simulink model "Final_Project_v3b"  (R2013a)
settings: Solver=ode45  StartTime=0.0  StopTime=inf  RelTol=1e-3
InitFcn:
  | start_EEVSCube2
  | 
  | %links masses
  | 
  | m=20;%Kg
  | 
  | l=1;%meter
  | 
  | %controls
  | 
  | a=0.3; %singularity positive gain
  | 
  | %Chaser
  | 
  | lb=1;%meter distance 1joint to CM
  | 
  | %Target
  | 
  | mt=5;%kg target mass
  | lt=1;%meter  side lenght
  | It=(1/6)*(lt^2);
  | 
  | %Target Initial Conitions
  | 
  | x_t=2;
  | y_t=3;
  | theta_t=0.7853;
  | 
  | Init_t=[x_t;y_t;theta_t];
undefined symbols (not defined in the file or in its folder): mesh_A, mesh_B
libraries: vrlib x2, dspinverses x1, aerolibanimutils x1
(part 1 of 2)
settings Model: Creator=Grompone  LastModifiedBy=Grompone

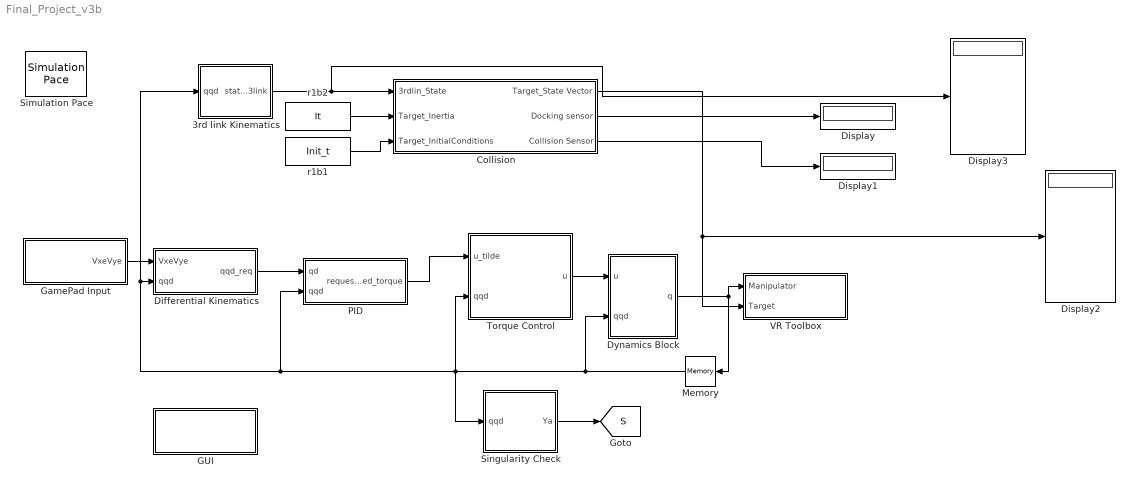
== system Final_Project_v3b ==
  3rd link Kinematics : MATLAB Function  TreatAsAtomicUnit=on
  Collision : Subsystem
  Differential Kinematics : Subsystem
  Display{,1..3} (4 alike) : Display
  Dynamics Block : Subsystem
  GUI : Subsystem
  GamePad Input : Subsystem
  Memory : Memory  X0=[0 0 0 0 0 0 0 0 0]'
  PID : Subsystem
  Simulation Pace : aerolibanimutils/Simulation Pace  SimulationPace=1  SleepMode=MATLAB Thread  OutputPaceError=off  SampleTime=1/30
      settings: AttributesFormatString=%<SimulationPace> sec/sec
  Singularity Check : MATLAB Function  TreatAsAtomicUnit=on
  Torque Control : Subsystem
  VR Toolbox : Subsystem
  r1b1 : Constant  Value=Init_t
  r1b2 : Constant  Value=It
  tag scope: S=global
  wires:
  Torque Control/1(u) -> Dynamics Block/1(u)
  PID/1(requested_torque) -> Torque Control/1(u_tilde)
  Dynamics Block/1(q) -> VR Toolbox/1(Manipulator), Memory/1
  Differential Kinematics/1(qqd_req) -> PID/1(qd)
  GamePad Input/1(VxeVye) -> Differential Kinematics/1(VxeVye)
  Memory/1 -> Dynamics Block/2(qqd), Torque Control/2(qqd), Singularity Check/1(qqd), PID/2(qqd), 3rd link Kinematics/1(qqd), Differential Kinematics/2(qqd)
  Singularity Check/1(Ya) -> [S]
  r1b2/1 -> Collision/2(Target_Inertia)
  r1b1/1 -> Collision/3(Target_InitialConditions)
  Collision/1(Target_State Vector) -> Display2/1, VR Toolbox/2(Target)
  3rd link Kinematics/1(state_3link) -> Display3/1, Collision/1(3rdlin_State)
  Collision/2(Docking sensor) -> Display/1
  Collision/3(Collision Sensor) -> Display1/1

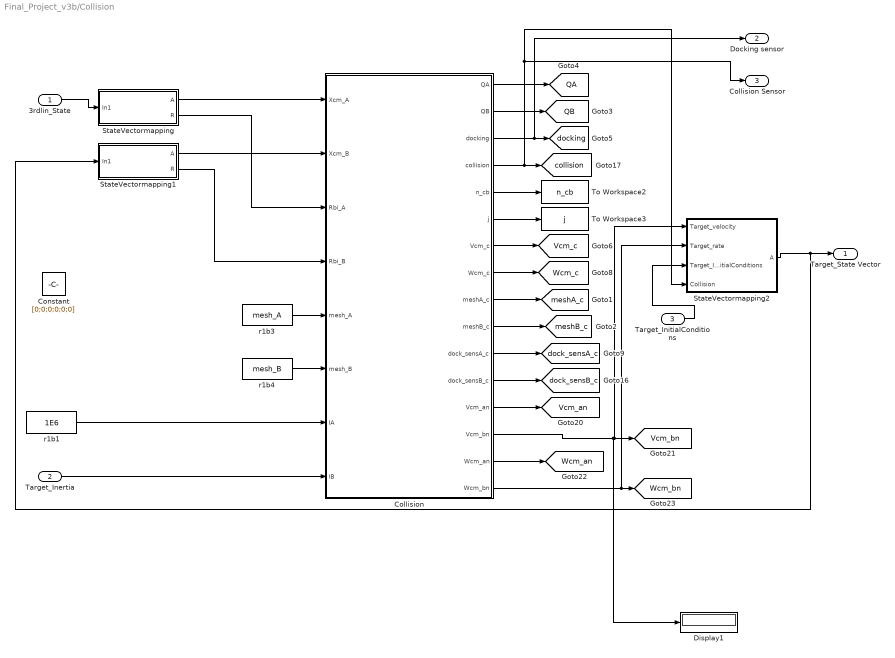
== system Final_Project_v3b/Collision ==
  3rdlin_State : Inport
  Target_Inertia : Inport  Port=2
  Target_InitialConditions : Inport  Port=3
  Collision : Subsystem  mask{mA=1e6, mB=mt, sigma=0.01, sigma_dock=0.1, dotsigma_dock=1, dock_sensA=[0.5 0 0]', dock_sensB=[-0.5 0 0]', epsilon=1}
      mask prompts: mA "Mass of body A [Kg]"; mB "Mass of body B [Kg]"; sigma "Minimum distance for contact [m]"; sigma_dock "Minimum distance for docking (must be greater than contact distance) [m]"; dotsigma_dock "Maximum relative velocity for docking [m/s]"; dock_sensA "Docking sensor position (Body RF) on body A (as [x y z]') [m]"; dock_sensB "Docking sensor position (Body RF) on body B (as [x y z]') [m]"; epsilon "Coefficent of restitution"
      mask help: This block implements collision detection and responce for two rigid bodies of general shapes.
      mask init:
      | ma_mb = [mA; 
      |          mB];
      mask Display:
      | image(imread('collision.jpeg'))
      | color('red');
      | disp('Collision \n Detection and Responce \n v.1.0.9')
      | port_label('input',1,'Xcm_A')
      | port_label('input',2,'Xcm_B')
      | port_label('input',3,'Rbi_A')
      | port_label('input',4,'Rbi_B')
      | port_label('input',5,'mesh_A')
      | port_label('input',6,'mesh_B')
      | port_label('input',7,'IA')
      | port_label('input',8,'IB')
      | 
      | port_label('output',1,'QA')
      | port_label('output',2,'QB')
      | port_label('output',3,'docking')
      | port_label('output',4,'collision')
      | port_label('output',5,'n_cb')
      | port_label('output',6,'j')
      | port_label('output',7,'Vcm_c')
      | port_label('output',8,'Wcm_c')
      | port_label('output',9,'meshA_c')
      | port_label('output',10,'meshB_c')
      | port_label('output',11,'dock_sensA_c')
      | port_label('output',12,'dock_sensB_c')
      | port_label('output',13,'Vcm_an')
      | port_label('output',14,'Vcm_bn')
      | port_label('output',15,'Wcm_an')
      | port_label('output',16,'Wcm_bn')
  Constant : Constant  Value=[0;0;0;0;0;0]
  Display1 : Display
  StateVectormapping : Subsystem
  StateVectormapping1 : Subsystem
  StateVectormapping2 : Subsystem
  To Workspace2 : ToWorkspace  VariableName=n_cb  SampleTime=-1
  To Workspace3 : ToWorkspace  VariableName=j  SampleTime=-1
  r1b1 : Constant  Value=1E6
  r1b3 : Constant  Value=mesh_A
  r1b4 : Constant  Value=mesh_B
  Target_State Vector : Outport
  Docking sensor : Outport  Port=2
  Collision Sensor : Outport  Port=3
  tag scope: QA=global, QB=global, Vcm_an=global, Vcm_bn=global, Vcm_c=global, Wcm_an=global, Wcm_bn=global, Wcm_c=global, collision=global, dock_sensA_c=global, dock_sensB_c=global, docking=global, meshA_c=global, meshB_c=global
  wires:
  Collision/1(QA) -> [QA]
  Collision/2(QB) -> [QB]
  Collision/3(docking) -> Docking sensor/1, [docking]
  Collision/6(j) -> To Workspace3/1
  Collision/4(collision) -> StateVectormapping2/4(Collision), Collision Sensor/1, [collision]
  StateVectormapping/2(R) -> Collision/3(Rbi_A)
  StateVectormapping1/2(R) -> Collision/4(Rbi_B)
  r1b3/1 -> Collision/5(mesh_A)
  r1b4/1 -> Collision/6(mesh_B)
  Collision/5(n_cb) -> To Workspace2/1
  Collision/7(Vcm_c) -> [Vcm_c]
  Collision/8(Wcm_c) -> [Wcm_c]
  Collision/9(meshA_c) -> [meshA_c]
  Collision/10(meshB_c) -> [meshB_c]
  Collision/11(dock_sensA_c) -> [dock_sensA_c]
  Collision/12(dock_sensB_c) -> [dock_sensB_c]
  r1b1/1 -> Collision/7(IA)
  Collision/13(Vcm_an) -> [Vcm_an]
  Collision/15(Wcm_an) -> [Wcm_an]
  Collision/16(Wcm_bn) -> StateVectormapping2/2(Target_rate), [Wcm_bn]
  3rdlin_State/1 -> StateVectormapping/1(In1)
  StateVectormapping1/1(A) -> Collision/2(Xcm_B)
  Collision/14(Vcm_bn) -> Display1/1, StateVectormapping2/1(Target_velocity), [Vcm_bn]
  Target_InitialConditions/1 -> StateVectormapping2/3(Target_InitialConditions)
  Target_Inertia/1 -> Collision/8(IB)
  StateVectormapping/1(A) -> Collision/1(Xcm_A)
  StateVectormapping2/1(A) -> StateVectormapping1/1(In1), Target_State Vector/1

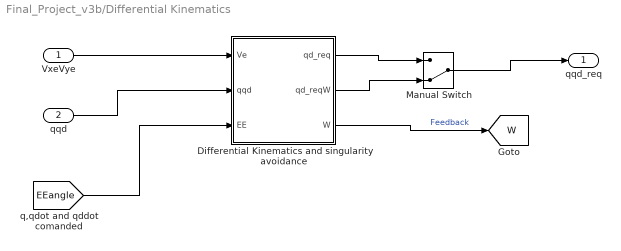
== system Final_Project_v3b/Differential Kinematics ==
  VxeVye : Inport
  qqd : Inport  Port=2
  Differential Kinematics and singularity avoidance : MATLAB Function  TreatAsAtomicUnit=on
  Manual Switch : ManualSwitch  CurrentSetting=0
  qqd_req : Outport
  tag scope: W=global
  wires:
  VxeVye/1 -> Differential Kinematics and singularity avoidance/1(Ve)
  qqd/1 -> Differential Kinematics and singularity avoidance/2(qqd)
  Differential Kinematics and singularity avoidance/3(W) -> [W]  "Feedback"
  Differential Kinematics and singularity avoidance/1(qd_req) -> Manual Switch/1
  Differential Kinematics and singularity avoidance/2(qd_reqW) -> Manual Switch/2
  Manual Switch/1 -> qqd_req/1
  [EEangle] -> Differential Kinematics and singularity avoidance/3(EE)

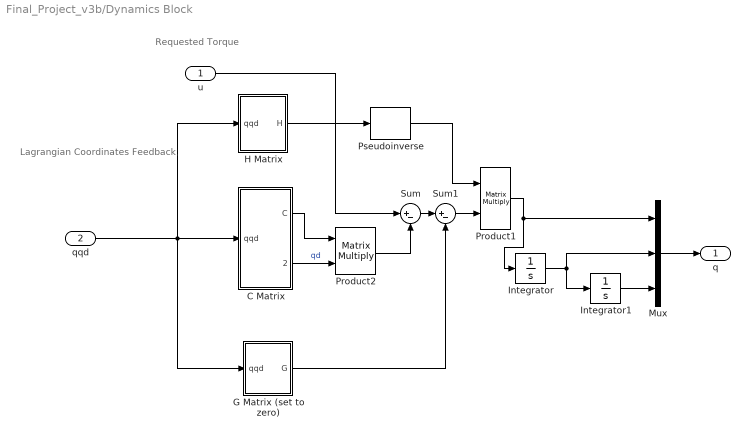
== system Final_Project_v3b/Dynamics Block ==
  note: Requested Torque
  note: Lagrangian Coordinates Feedback
  u : Inport
  qqd : Inport  Port=2
  C Matrix : MATLAB Function  TreatAsAtomicUnit=on
  G Matrix (set to zero) : MATLAB Function  TreatAsAtomicUnit=on
  H Matrix : MATLAB Function  TreatAsAtomicUnit=on
  Integrator : Integrator  InitialCondition=[0;0;0]
  Integrator1 : Integrator  InitialCondition=[0;0;0]
  Mux : Mux  Inputs=3
  Product1 : Product  Multiplication=Matrix(*)
  Product2 : Product  Multiplication=Matrix(*)  OutDataTypeStr=int8  LockScale=on
  Pseudoinverse : dspinverses/Pseudoinverse  wanterr=off
  Sum : Sum  Inputs=|+-
  Sum1 : Sum  Inputs=|+-
  q : Outport
  wires:
  Integrator/1 -> Mux/2, Integrator1/1
  Integrator1/1 -> Mux/3
  Mux/1 -> q/1
  C Matrix/1(C) -> Product2/1
  H Matrix/1(H) -> Pseudoinverse/1
  Pseudoinverse/1 -> Product1/1
  Product1/1 -> Mux/1, Integrator/1
  Sum/1 -> Sum1/1
  Sum1/1 -> Product1/2
  G Matrix (set to zero)/1(G) -> Sum1/2
  Product2/1 -> Sum/2
  u/1 -> Sum/1
  C Matrix/2(q_dot) -> Product2/2  "qd"
  qqd/1 -> G Matrix (set to zero)/1(qqd), H Matrix/1(qqd), C Matrix/1(qqd)

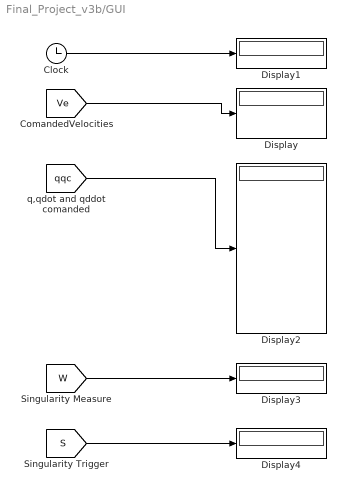
== system Final_Project_v3b/GUI ==
  Clock : Clock
  Display{,1..4} (5 alike) : Display
  wires:
  [Ve] -> Display/1
  Clock/1 -> Display1/1
  [qqc] -> Display2/1
  [W] -> Display3/1
  [S] -> Display4/1

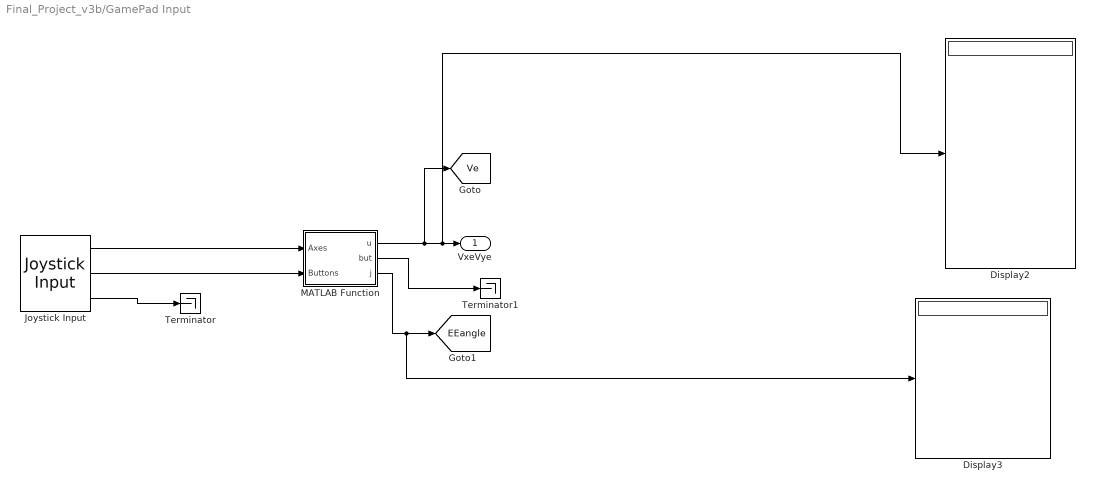
== system Final_Project_v3b/GamePad Input ==
  Display2 : Display
  Display3 : Display
  Joystick Input : vrlib/Joystick Input  joyid=1  adjustports=on  forcefeed=off
  MATLAB Function : MATLAB Function  TreatAsAtomicUnit=on
  Terminator : Terminator
  Terminator1 : Terminator
  VxeVye : Outport
  tag scope: EEangle=global, Ve=global
  wires:
  Joystick Input/1 -> MATLAB Function/1(Axes)
  Joystick Input/2 -> MATLAB Function/2(Buttons)
  MATLAB Function/1(u) -> [Ve], Display2/1, VxeVye/1
  Joystick Input/3 -> Terminator/1
  MATLAB Function/2(but) -> Terminator1/1
  MATLAB Function/3(j) -> Display3/1, [EEangle]

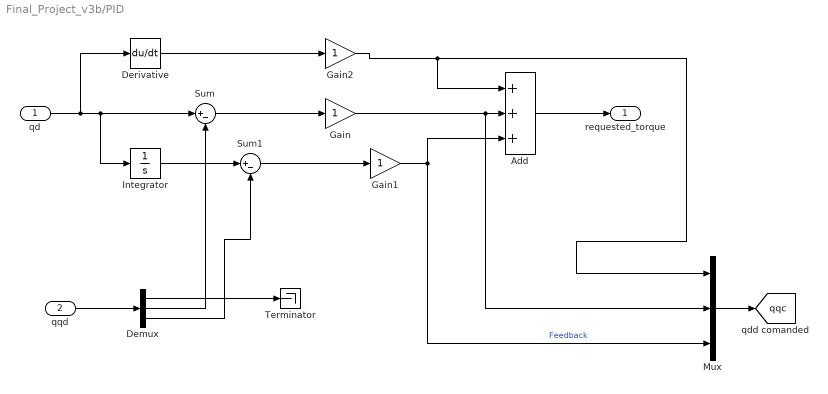
== system Final_Project_v3b/PID ==
  qd : Inport
  qqd : Inport  Port=2
  Add : Sum  Inputs=+++
  Demux : Demux  Outputs=3
  Derivative : Derivative
  Gain : Gain
  Gain1 : Gain
  Gain2 : Gain
  Integrator : Integrator  InitialCondition=[0; 0; 0]
  Mux : Mux  Inputs=3
  Sum : Sum  Inputs=|+-
  Sum1 : Sum  Inputs=|+-
  Terminator : Terminator
  requested_torque : Outport
  tag scope: qqc=global
  wires:
  qqd/1 -> Demux/1
  Demux/2 -> Sum/2
  Demux/1 -> Terminator/1
  Sum/1 -> Gain/1
  qd/1 -> Derivative/1, Integrator/1, Sum/1
  Gain/1 -> Mux/2, Add/2
  Sum1/1 -> Gain1/1
  Demux/3 -> Sum1/2
  Add/1 -> requested_torque/1
  Mux/1 -> [qqc]
  Gain1/1 -> Mux/3, Add/3  "Feedback"
  Integrator/1 -> Sum1/1
  Gain2/1 -> Add/1, Mux/1
  Derivative/1 -> Gain2/1

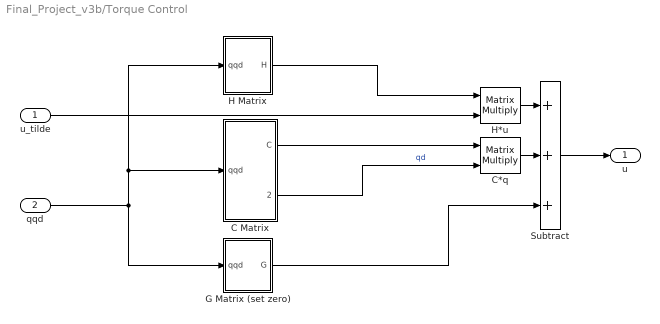
== system Final_Project_v3b/Torque Control ==
  u_tilde : Inport
  qqd : Inport  Port=2
  C Matrix : MATLAB Function  TreatAsAtomicUnit=on
  C*q : Product  Multiplication=Matrix(*)
  G Matrix (set zero) : MATLAB Function  TreatAsAtomicUnit=on
  H Matrix : MATLAB Function  TreatAsAtomicUnit=on
  H*u : Product  Multiplication=Matrix(*)
  Subtract : Sum  Inputs=+++
  u : Outport
  wires:
  H*u/1 -> Subtract/1
  Subtract/1 -> u/1
  C*q/1 -> Subtract/2
  C Matrix/1(C) -> C*q/1
  G Matrix (set zero)/1(G) -> Subtract/3
  C Matrix/2(q_dot) -> C*q/2  "qd"
  u_tilde/1 -> H*u/2
  H Matrix/1(H) -> H*u/1
  qqd/1 -> H Matrix/1(qqd), C Matrix/1(qqd), G Matrix (set zero)/1(qqd)

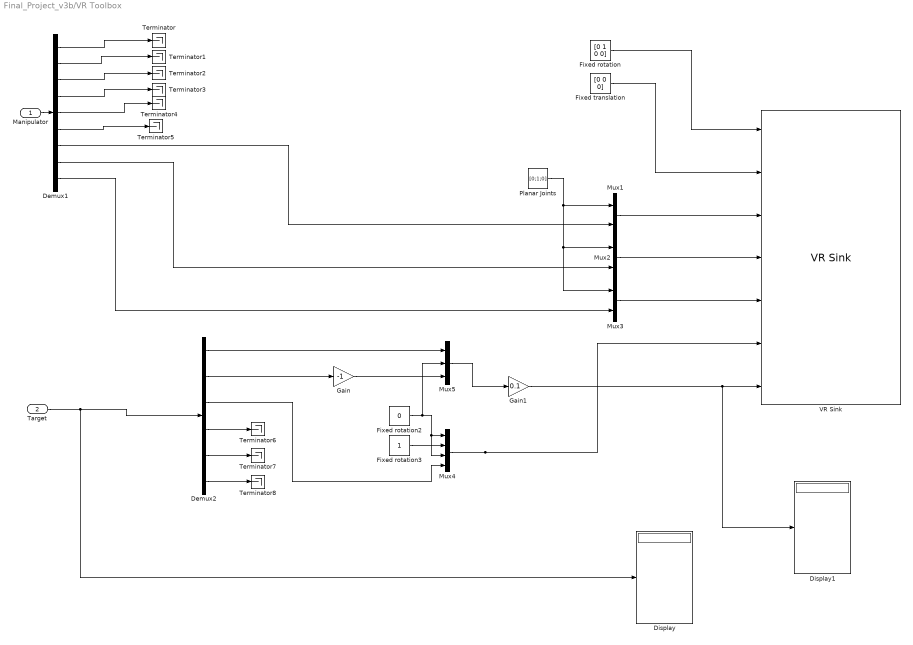
== system Final_Project_v3b/VR Toolbox ==
  Manipulator : Inport
  Target : Inport  Port=2
  Demux1 : Demux  Outputs=9
  Demux2 : Demux  Outputs=6
  Display : Display
  Display1 : Display
  Fixed rotation : Constant  Value=[0 1 0 0]
  Fixed rotation2 : Constant  Value=0
  Fixed rotation3 : Constant
  Fixed translation : Constant  Value=[0 0 0]
  Gain : Gain  Gain=-1
  Gain1 : Gain  Gain=0.1
  Mux1 : Mux  Inputs=2
  Mux2 : Mux  Inputs=2
  Mux3 : Mux  Inputs=2
  Mux4 : Mux
  Mux5 : Mux  Inputs=3
  Planar Joints : Constant  Value=[0;1;0]
  Terminator{,1..8} (9 alike) : Terminator
  VR Sink : vrlib/VR Sink  InstantiateOnLoad=on  SampleTime=0.1  ViewEnable=on  RemoteChange=off  RemoteView=off  FieldsWritten=CHASER.rotation.4.1.1.double#CHASER.translation.3.1.1.double#Joint1.rotation.4.1.1.double#Joint2.rotation.4.1.1.double#Joint3.rotation.4.1.1.double#TARGET.rotation.4.1.1.double#TARGET.translation.3.1.1.double  WorldFileName=final1.wrl  AutoView=off  VideoDimensions=[]  AllowVariableSize=off  FigureProperties="{'Position', 'Name', 'Viewpoint', 'CameraBound', 'CameraDirection', 'CameraPosition', 'CameraUpVector', 'ZoomFactor', 'Antialiasing', 'Headlight', 'Lighting', 'NavPanel', 'StatusBar', 'ToolBar', 'Textures', 'Transparency', 'Triad', 'Wireframe', 'NavZones', 'NavMode', 'NavSpeed', 'CaptureFileFormat', 'CaptureFileName', 'Record2DCompressMethod', 'Record2DCompressQuality', 'Record2D', 'Record2DFileName', 'Record2DFPS'; [5.0000000000000000e+00   9.2000000000000000e+01   5.7600000000000000e+02   3.8000000000000000e+02], '', '_untitled_1', 'on', [0.0000000000000000e+00   0.0000000000000000e+00  -1.0000000000000000e+00], [0.0000000000000000e+00   0.0000000000000000e+00   0.0000000000000000e+00], [0.0000000000000000e+00   1.0000000000000000e+00   0.0000000000000000e+00], [1.0000000000000000e+00], 'on', 'on', 'on', 'halfbar', 'on', 'on', 'on', 'on', 'none', 'off', 'off', 'fly', 'normal', 'tif', '%f_anim_%n.tif', 'auto', [7.5000000000000000e+01], 'off', '%f_anim_%n.avi', [1.5000000000000000e+01]}"
  wires:
  Planar Joints/1 -> Mux3/1, Mux2/1, Mux1/1
  Manipulator/1 -> Demux1/1
  Demux1/8 -> Mux2/2
  Demux1/9 -> Mux3/2
  Demux1/7 -> Mux1/2
  Demux1/1 -> Terminator/1
  Demux1/2 -> Terminator1/1
  Demux1/3 -> Terminator2/1
  Demux1/4 -> Terminator3/1
  Demux1/5 -> Terminator4/1
  Demux1/6 -> Terminator5/1
  Fixed rotation/1 -> VR Sink/1
  Fixed translation/1 -> VR Sink/2
  Mux1/1 -> VR Sink/3
  Mux2/1 -> VR Sink/4
  Mux3/1 -> VR Sink/5
  Target/1 -> Display/1, Demux2/1
  Fixed rotation3/1 -> Mux4/2
  Fixed rotation2/1 -> Mux5/2, Mux4/3, Mux4/1
  Demux2/1 -> Mux5/1
  Demux2/2 -> Gain/1
  Demux2/3 -> Mux4/4
  Demux2/4 -> Terminator6/1
  Demux2/5 -> Terminator7/1
  Demux2/6 -> Terminator8/1
  Gain/1 -> Mux5/3
  Mux4/1 -> VR Sink/6
  Mux5/1 -> Gain1/1
  Gain1/1 -> Display1/1, VR Sink/7

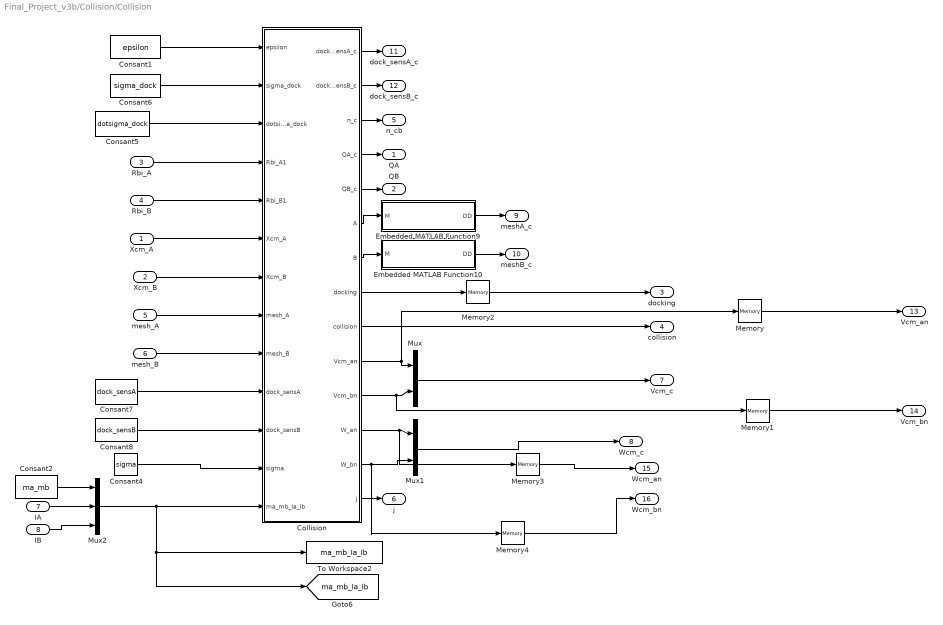
== system Final_Project_v3b/Collision/Collision ==
  Xcm_A : Inport
  Xcm_B : Inport  Port=2
  Rbi_A : Inport  Port=3
  Rbi_B : Inport  Port=4
  mesh_A : Inport  Port=5
  mesh_B : Inport  Port=6
  IA : Inport  Port=7
  IB : Inport  Port=8
  Collision : MATLAB Function  TreatAsAtomicUnit=on
  Consant1 : Constant  Value=epsilon
  Consant2 : Constant  Value=ma_mb
  Consant4 : Constant  Value=sigma
  Consant5 : Constant  Value=dotsigma_dock
  Consant6 : Constant  Value=sigma_dock
  Consant7 : Constant  Value=dock_sensA
  Consant8 : Constant  Value=dock_sensB
  Embedded MATLAB Function10 : MATLAB Function  TreatAsAtomicUnit=on
  Embedded MATLAB Function9 : MATLAB Function  TreatAsAtomicUnit=on
  Memory{,1,3..4} (4 alike) : Memory  X0=zeros(3,1)
  Memory2 : Memory
  Mux : Mux  Inputs=2
  Mux1 : Mux  Inputs=2
  Mux2 : Mux  Inputs=3
  To Workspace2 : ToWorkspace  VariableName=ma_mb_Ia_Ib  SampleTime=-1
  QA : Outport
  QB : Outport  Port=2
  docking : Outport  Port=3
  collision : Outport  Port=4
  n_cb : Outport  Port=5
  j : Outport  Port=6
  Vcm_c : Outport  Port=7
  Wcm_c : Outport  Port=8
  meshA_c : Outport  Port=9
  meshB_c : Outport  Port=10
  dock_sensA_c : Outport  Port=11
  dock_sensB_c : Outport  Port=12
  Vcm_an : Outport  Port=13
  Vcm_bn : Outport  Port=14
  Wcm_an : Outport  Port=15
  Wcm_bn : Outport  Port=16
  tag scope: ma_mb_Ia_Ib=global
  wires:
  Embedded MATLAB Function9/1(DD) -> meshA_c/1
  Embedded MATLAB Function10/1(DD) -> meshB_c/1
  Collision/6(A) -> Embedded MATLAB Function9/1(M)
  Collision/7(B) -> Embedded MATLAB Function10/1(M)
  Rbi_B/1 -> Collision/5(Rbi_B1)
  Xcm_A/1 -> Collision/6(Xcm_A)
  mesh_A/1 -> Collision/8(mesh_A)
  mesh_B/1 -> Collision/9(mesh_B)
  Collision/3(n_c) -> n_cb/1
  Collision/8(docking) -> Memory2/1
  Collision/10(Vcm_an) -> Mux/1, Memory/1
  Collision/13(W_bn) -> Mux1/2, Memory4/1
  Collision/14(j) -> j/1
  Collision/9(collision) -> collision/1
  Mux/1 -> Vcm_c/1
  Mux1/1 -> Wcm_c/1
  Collision/4(QA_c) -> QA/1
  Collision/5(QB_c) -> QB/1
  Collision/11(Vcm_bn) -> Memory1/1, Mux/2
  Collision/12(W_an) -> Memory3/1, Mux1/1
  Xcm_B/1 -> Collision/7(Xcm_B)
  Collision/2(dock_sensB_c) -> dock_sensB_c/1
  Collision/1(dock_sensA_c) -> dock_sensA_c/1
  Consant4/1 -> Collision/12(sigma)
  Consant5/1 -> Collision/3(dotsigma_dock)
  Rbi_A/1 -> Collision/4(Rbi_A1)
  Consant6/1 -> Collision/2(sigma_dock)
  Consant7/1 -> Collision/10(dock_sensA)
  Consant8/1 -> Collision/11(dock_sensB)
  Consant1/1 -> Collision/1(epsilon)
  Mux2/1 -> Collision/13(ma_mb_Ia_Ib), To Workspace2/1, [ma_mb_Ia_Ib]
  Consant2/1 -> Mux2/1
  IA/1 -> Mux2/2
  IB/1 -> Mux2/3
  Memory/1 -> Vcm_an/1
  Memory1/1 -> Vcm_bn/1
  Memory3/1 -> Wcm_an/1
  Memory4/1 -> Wcm_bn/1
  Memory2/1 -> docking/1

== system Final_Project_v3b/Collision/StateVectormapping ==
  In1 : Inport
  Rotation MAtrix1 : MATLAB Function  TreatAsAtomicUnit=on
  A : Outport
  R : Outport  Port=2
  wires:
  Rotation MAtrix1/2(R) -> R/1
  In1/1 -> Rotation MAtrix1/1(u)
  Rotation MAtrix1/1(y) -> A/1

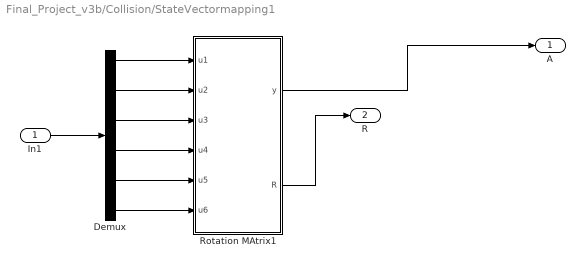
== system Final_Project_v3b/Collision/StateVectormapping1 ==
  In1 : Inport
  Demux : Demux  Outputs=6
  Rotation MAtrix1 : MATLAB Function  TreatAsAtomicUnit=on
  A : Outport  PortDimensions=[9,1]
  R : Outport  Port=2
  wires:
  Demux/1 -> Rotation MAtrix1/1(u1)
  Demux/2 -> Rotation MAtrix1/2(u2)
  Demux/3 -> Rotation MAtrix1/3(u3)
  Demux/6 -> Rotation MAtrix1/6(u6)
  Demux/4 -> Rotation MAtrix1/4(u4)
  Demux/5 -> Rotation MAtrix1/5(u5)
  In1/1 -> Demux/1
  Rotation MAtrix1/2(R) -> R/1
  Rotation MAtrix1/1(y) -> A/1

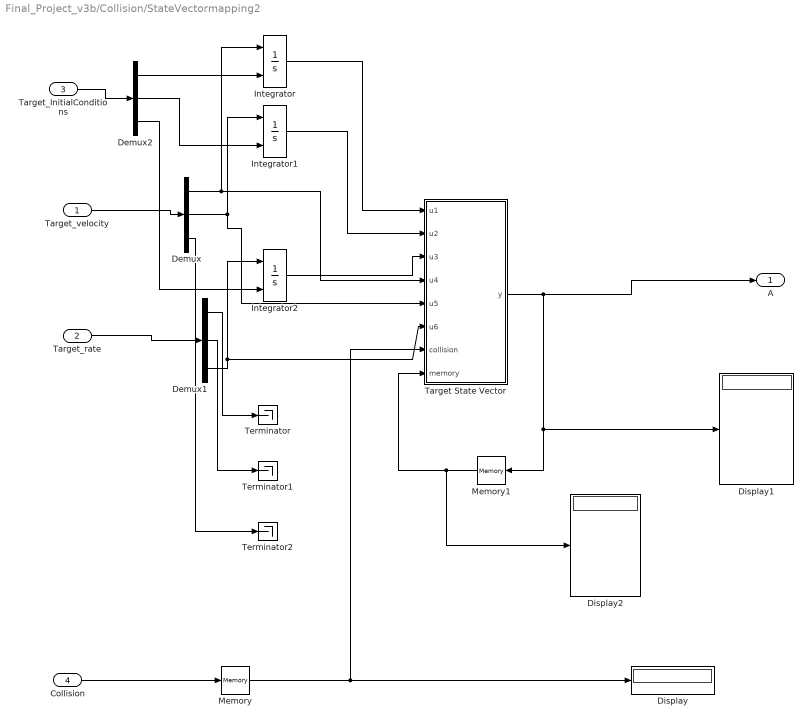
== system Final_Project_v3b/Collision/StateVectormapping2 ==
  Target_velocity : Inport
  Target_rate : Inport  Port=2
  Target_InitialConditions : Inport  Port=3
  Collision : Inport  Port=4
  Demux : Demux  Outputs=3
  Demux1 : Demux  Outputs=3
  Demux2 : Demux  Outputs=3
  Display : Display
  Display1 : Display
  Display2 : Display
  Integrator : Integrator  InitialConditionSource=external
  Integrator1 : Integrator  InitialConditionSource=external
  Integrator2 : Integrator  InitialConditionSource=external
  Memory : Memory  X0=1
  Memory1 : Memory  X0=[0 0 0 0 0 0]'
  Target State Vector : MATLAB Function  TreatAsAtomicUnit=on
  Terminator : Terminator
  Terminator1 : Terminator
  Terminator2 : Terminator
  A : Outport
  wires:
  Target_velocity/1 -> Demux/1
  Target_rate/1 -> Demux1/1
  Demux1/3 -> Integrator2/1, Target State Vector/6(u6)
  Demux/2 -> Target State Vector/5(u5), Integrator1/1
  Demux/1 -> Target State Vector/4(u4), Integrator/1
  Integrator/1 -> Target State Vector/1(u1)
  Integrator1/1 -> Target State Vector/2(u2)
  Integrator2/1 -> Target State Vector/3(u3)
  Demux1/2 -> Terminator1/1
  Demux1/1 -> Terminator/1
  Target_InitialConditions/1 -> Demux2/1
  Demux2/1 -> Integrator/2
  Demux2/2 -> Integrator1/2
  Demux2/3 -> Integrator2/2
  Demux/3 -> Terminator2/1
  Target State Vector/1(y) -> Display1/1, Memory1/1, A/1
  Collision/1 -> Memory/1
  Memory1/1 -> Display2/1, Target State Vector/8(memory)
  Memory/1 -> Target State Vector/7(collision), Display/1

== matlab function Final_Project_v3b/Dynamics Block/C Matrix ==
  data: qqd input; C output; m parameter; l parameter; q_dot output
function [C,q_dot] = fcn(qqd,m,l)
q=[qqd(7); qqd(8); qqd(9)];
q_dot=[qqd(4); qqd(5); qqd(6)];
C=[                                                                                                                                                                                                                                                                                                                                                                                                                                                                                                                                                  (m*abs(l)^2*(2*sin(conj(q(1))) + sin(conj(q(1)) + conj(q(2)) + conj(q(3))) + 2*sin(conj(q(1)) + conj(q(2))))*(cos(q(1) + q(2) + q(3))*(q_dot(1) + q_dot(2) + q_dot(3)) + 2*cos(q(1) + q(2))*(q_dot(1) + q_dot(2)) + 2*q_dot(1)*cos(q(1))))/8 - (m*abs(l)^2*(2*cos(conj(q(1))) + cos(conj(q(1)) + conj(q(2)) + conj(q(3))) + 2*cos(conj(q(1)) + conj(q(2))))*(sin(q(1) + q(2) + q(3))*(q_dot(1) + q_dot(2) + q_dot(3)) + 2*sin(q(1) + q(2))*(q_dot(1) + q_dot(2)) + 2*q_dot(1)*sin(q(1))))/8 + (m*abs(l)^2*(cos(q(1) + q(2))*(q_dot(1) + q_dot(2)) + 2*q_dot(1)*cos(q(1)))*(2*sin(conj(q(1))) + sin(conj(q(1)) + conj(q(2)))))/8 - (m*abs(l)^2*(2*cos(conj(q(1))) + cos(conj(q(1)) + conj(q(2))))*(sin(q(1) + q(2))*(q_dot(1) + q_dot(2)) + 2*q_dot(1)*sin(q(1))))/8 - (m*abs(l)^2*(cos(q(1) + q(2)) + 2*cos(q(1)))*(2*sin(conj(q(1)))*conj(q_dot(1)) + sin(conj(q(1)) + conj(q(2)))*(conj(q_dot(1)) + conj(q_dot(2)))))/8 + (m*abs(l)^2*(sin(q(1) + q(2)) + 2*sin(q(1)))*(2*cos(conj(q(1)))*conj(q_dot(1)) + cos(conj(q(1)) + conj(q(2)))*(conj(q_dot(1)) + conj(q_dot(2)))))/8 + (m*abs(l)^2*(2*cos(conj(q(1)))*conj(q_dot(1)) + cos(conj(q(1)) + conj(q(2)) + conj(q(3)))*(conj(q_dot(1)) + conj(q_dot(2)) + conj(q_dot(3))) + 2*cos(conj(q(1)) + conj(q(2)))*(conj(q_dot(1)) + conj(q_dot(2))))*(sin(q(1) + q(2) + q(3)) + 2*sin(q(1) + q(2)) + 2*sin(q(1))))/8 - (m*abs(l)^2*(2*sin(conj(q(1)))*conj(q_dot(1)) + sin(conj(q(1)) + conj(q(2)) + conj(q(3)))*(conj(q_dot(1)) + conj(q_dot(2)) + conj(q_dot(3))) + 2*sin(conj(q(1)) + conj(q(2)))*(conj(q_dot(1)) + conj(q_dot(2))))*(cos(q(1) + q(2) + q(3)) + 2*cos(q(1) + q(2)) + 2*cos(q(1))))/8 - (m*q_dot(1)*cos(conj(q(1)))*abs(l)^2*sin(q(1)))/8 + (m*q_dot(1)*sin(conj(q(1)))*abs(l)^2*cos(q(1)))/8 + (m*cos(conj(q(1)))*abs(l)^2*conj(q_dot(1))*sin(q(1)))/8 - (m*sin(conj(q(1)))*abs(l)^2*cos(q(1))*conj(q_dot(1)))/8,                                                                                                                                                                                                                                     (m*sin(conj(q(1)) - q(2) - q(3) - q(1))*abs(l)^2)/2 + (3*m*sin(conj(q(1)) - q(2) - q(1))*abs(l)^2)/4 + (m*abs(l)^2*sin(conj(q(1)) - q(2) - q(3) - q(1) + conj(q(2)))*(q_dot(1) + q_dot(2) + q_dot(3) - conj(q_dot(1)) - conj(q_dot(2))))/4 + (m*sin(conj(q(1)) - q(2) - q(3) - q(1) + conj(q(2)) + conj(q(3)))*abs(l)^2*(q_dot(1) + q_dot(2) + q_dot(3) - conj(q_dot(1)) - conj(q_dot(2)) - conj(q_dot(3))))/8 - (m*sin(q(1) + q(2))*abs(l)^2*(2*cos(conj(q(1))) + cos(conj(q(1)) + conj(q(2)))))/8 + (m*cos(q(1) + q(2))*abs(l)^2*(2*sin(conj(q(1))) + sin(conj(q(1)) + conj(q(2)))))/8 - (m*abs(l)^2*(sin(conj(q(1)) + conj(q(2)) + conj(q(3))) + 2*sin(conj(q(1)) + conj(q(2))))*(cos(q(1) + q(2) + q(3)) + 2*cos(q(1) + q(2)) + 2*cos(q(1))))/8 + (m*abs(l)^2*(cos(conj(q(1)) + conj(q(2)) + conj(q(3))) + 2*cos(conj(q(1)) + conj(q(2))))*(sin(q(1) + q(2) + q(3)) + 2*sin(q(1) + q(2)) + 2*sin(q(1))))/8 - (m*abs(l)^2*sin(conj(q(1)) - q(2) - q(1) + conj(q(2)) + conj(q(3)))*(conj(q_dot(1)) - q_dot(2) - q_dot(1) + conj(q_dot(2)) + conj(q_dot(3))))/4 - (m*abs(l)^2*(sin(q(1) + q(2) + q(3)) + 2*sin(q(1) + q(2)))*(2*cos(conj(q(1))) + cos(conj(q(1)) + conj(q(2)) + conj(q(3))) + 2*cos(conj(q(1)) + conj(q(2)))))/8 + (m*abs(l)^2*(cos(q(1) + q(2) + q(3)) + 2*cos(q(1) + q(2)))*(2*sin(conj(q(1))) + sin(conj(q(1)) + conj(q(2)) + conj(q(3))) + 2*sin(conj(q(1)) + conj(q(2)))))/8 - (m*sin(conj(q(1)) + conj(q(2)))*abs(l)^2*(cos(q(1) + q(2)) + 2*cos(q(1))))/8 + (3*m*sin(conj(q(1)) - q(2) - q(1))*abs(l)^2*(q_dot(1) + q_dot(2) - conj(q_dot(1))))/4 + (m*cos(conj(q(1)) + conj(q(2)))*abs(l)^2*(sin(q(1) + q(2)) + 2*sin(q(1))))/8 + (5*m*sin(conj(q(1)) - q(2) - q(1) + conj(q(2)))*abs(l)^2*(q_dot(1) + q_dot(2) - conj(q_dot(1)) - conj(q_dot(2))))/8 + (m*sin(conj(q(1)) - q(2) - q(3) - q(1))*abs(l)^2*(q_dot(1) + q_dot(2) + q_dot(3) - conj(q_dot(1))))/4, (m*sin(conj(q(1)) - q(2) - q(3) - q(1))*abs(l)^2)/4 + (m*abs(l)^2*(2*sin(conj(q(1)) - q(2) - q(3) - q(1)) + 2*sin(conj(q(1)) - q(2) - q(3) - q(1) + conj(q(2)))))/8 + (m*abs(l)^2*(2*sin(conj(q(1)) - q(2) - q(3) - q(1))*(q_dot(1) + q_dot(2) + q_dot(3) - conj(q_dot(1))) + 2*sin(conj(q(1)) - q(2) - q(3) - q(1) + conj(q(2)))*(q_dot(1) + q_dot(2) + q_dot(3) - conj(q_dot(1)) - conj(q_dot(2))) + sin(conj(q(1)) - q(2) - q(3) - q(1) + conj(q(2)) + conj(q(3)))*(q_dot(1) + q_dot(2) + q_dot(3) - conj(q_dot(1)) - conj(q_dot(2)) - conj(q_dot(3)))))/8 + (m*abs(l)^2*sin(conj(q(1)) - q(2) - q(3) - q(1) + conj(q(2))))/4 - (m*abs(l)^2*sin(conj(q(1)) - q(2) - q(1) + conj(q(2)) + conj(q(3))))/4 + (m*cos(conj(q(1)) + conj(q(2)) + conj(q(3)))*abs(l)^2*(sin(q(1) + q(2) + q(3)) + 2*sin(q(1) + q(2)) + 2*sin(q(1))))/8 - (m*sin(q(1) + q(2) + q(3))*abs(l)^2*(2*cos(conj(q(1))) + cos(conj(q(1)) + conj(q(2)) + conj(q(3))) + 2*cos(conj(q(1)) + conj(q(2)))))/8 + (m*cos(q(1) + q(2) + q(3))*abs(l)^2*(2*sin(conj(q(1))) + sin(conj(q(1)) + conj(q(2)) + conj(q(3))) + 2*sin(conj(q(1)) + conj(q(2)))))/8 - (m*sin(conj(q(1)) + conj(q(2)) + conj(q(3)))*abs(l)^2*(cos(q(1) + q(2) + q(3)) + 2*cos(q(1) + q(2)) + 2*cos(q(1))))/8;
 (m*sin(conj(q(1)) - q(2) - q(3) - q(1))*abs(l)^2)/2 + (3*m*sin(conj(q(1)) - q(2) - q(1))*abs(l)^2)/4 - (m*abs(l)^2*(cos(conj(q(1)) + conj(q(2)) + conj(q(3))) + 2*cos(conj(q(1)) + conj(q(2))))*(sin(q(1) + q(2) + q(3))*(q_dot(1) + q_dot(2) + q_dot(3)) + 2*sin(q(1) + q(2))*(q_dot(1) + q_dot(2)) + 2*q_dot(1)*sin(q(1))))/8 - (m*sin(q(1) + q(2))*abs(l)^2*(2*cos(conj(q(1))) + cos(conj(q(1)) + conj(q(2)))))/8 + (m*cos(q(1) + q(2))*abs(l)^2*(2*sin(conj(q(1))) + sin(conj(q(1)) + conj(q(2)))))/8 - (m*abs(l)^2*(sin(conj(q(1)) + conj(q(2)) + conj(q(3))) + 2*sin(conj(q(1)) + conj(q(2))))*(cos(q(1) + q(2) + q(3)) + 2*cos(q(1) + q(2)) + 2*cos(q(1))))/8 + (m*abs(l)^2*(cos(conj(q(1)) + conj(q(2)) + conj(q(3))) + 2*cos(conj(q(1)) + conj(q(2))))*(sin(q(1) + q(2) + q(3)) + 2*sin(q(1) + q(2)) + 2*sin(q(1))))/8 - (m*abs(l)^2*(sin(conj(q(1)) + conj(q(2)) + conj(q(3)))*(conj(q_dot(1)) + conj(q_dot(2)) + conj(q_dot(3))) + 2*sin(conj(q(1)) + conj(q(2)))*(conj(q_dot(1)) + conj(q_dot(2))))*(cos(q(1) + q(2) + q(3)) + 2*cos(q(1) + q(2)) + 2*cos(q(1))))/8 + (m*abs(l)^2*(cos(conj(q(1)) + conj(q(2)) + conj(q(3)))*(conj(q_dot(1)) + conj(q_dot(2)) + conj(q_dot(3))) + 2*cos(conj(q(1)) + conj(q(2)))*(conj(q_dot(1)) + conj(q_dot(2))))*(sin(q(1) + q(2) + q(3)) + 2*sin(q(1) + q(2)) + 2*sin(q(1))))/8 - (m*abs(l)^2*(sin(q(1) + q(2) + q(3)) + 2*sin(q(1) + q(2)))*(2*cos(conj(q(1))) + cos(conj(q(1)) + conj(q(2)) + conj(q(3))) + 2*cos(conj(q(1)) + conj(q(2)))))/8 + (m*abs(l)^2*(cos(q(1) + q(2) + q(3)) + 2*cos(q(1) + q(2)))*(2*sin(conj(q(1))) + sin(conj(q(1)) + conj(q(2)) + conj(q(3))) + 2*sin(conj(q(1)) + conj(q(2)))))/8 - (m*sin(conj(q(1)) + conj(q(2)))*abs(l)^2*(cos(q(1) + q(2)) + 2*cos(q(1))))/8 + (m*cos(conj(q(1)) + conj(q(2)))*abs(l)^2*(sin(q(1) + q(2)) + 2*sin(q(1))))/8 + (m*sin(conj(q(1)) + conj(q(2)))*abs(l)^2*(cos(q(1) + q(2))*(q_dot(1) + q_dot(2)) + 2*q_dot(1)*cos(q(1))))/8 - (m*cos(conj(q(1)) + conj(q(2)))*abs(l)^2*(sin(q(1) + q(2))*(q_dot(1) + q_dot(2)) + 2*q_dot(1)*sin(q(1))))/8 + (m*abs(l)^2*(sin(conj(q(1)) + conj(q(2)) + conj(q(3))) + 2*sin(conj(q(1)) + conj(q(2))))*(cos(q(1) + q(2) + q(3))*(q_dot(1) + q_dot(2) + q_dot(3)) + 2*cos(q(1) + q(2))*(q_dot(1) + q_dot(2)) + 2*q_dot(1)*cos(q(1))))/8 - (m*sin(conj(q(1)) + conj(q(2)))*abs(l)^2*(conj(q_dot(1)) + conj(q_dot(2)))*(cos(q(1) + q(2)) + 2*cos(q(1))))/8 + (m*cos(conj(q(1)) + conj(q(2)))*abs(l)^2*(conj(q_dot(1)) + conj(q_dot(2)))*(sin(q(1) + q(2)) + 2*sin(q(1))))/8, (m*sin(conj(q(1)) + conj(q(2)))*cos(q(1) + q(2))*abs(l)^2)/4 - (m*cos(conj(q(1)) + conj(q(2)))*sin(q(1) + q(2))*abs(l)^2)/4 - (m*abs(l)^2*(sin(conj(q(1)) + conj(q(2)) + conj(q(3))) + 2*sin(conj(q(1)) + conj(q(2))))*(cos(q(1) + q(2) + q(3)) + 2*cos(q(1) + q(2)) + 2*cos(q(1))))/4 + (m*abs(l)^2*(cos(conj(q(1)) + conj(q(2)) + conj(q(3))) + 2*cos(conj(q(1)) + conj(q(2))))*(sin(q(1) + q(2) + q(3)) + 2*sin(q(1) + q(2)) + 2*sin(q(1))))/4 - (m*abs(l)^2*(cos(q(1) + q(2) + q(3)) + 2*cos(q(1) + q(2)))*(sin(conj(q(1)) + conj(q(2)) + conj(q(3)))*(conj(q_dot(1)) + conj(q_dot(2)) + conj(q_dot(3))) + 2*sin(conj(q(1)) + conj(q(2)))*(conj(q_dot(1)) + conj(q_dot(2)))))/8 + (m*abs(l)^2*(sin(q(1) + q(2) + q(3)) + 2*sin(q(1) + q(2)))*(cos(conj(q(1)) + conj(q(2)) + conj(q(3)))*(conj(q_dot(1)) + conj(q_dot(2)) + conj(q_dot(3))) + 2*cos(conj(q(1)) + conj(q(2)))*(conj(q_dot(1)) + conj(q_dot(2)))))/8 - (m*abs(l)^2*(cos(conj(q(1)) + conj(q(2)) + conj(q(3))) + 2*cos(conj(q(1)) + conj(q(2))))*(sin(q(1) + q(2) + q(3))*(q_dot(1) + q_dot(2) + q_dot(3)) + 2*sin(q(1) + q(2))*(q_dot(1) + q_dot(2))))/8 + (m*abs(l)^2*(sin(conj(q(1)) + conj(q(2)) + conj(q(3))) + 2*sin(conj(q(1)) + conj(q(2))))*(cos(q(1) + q(2) + q(3))*(q_dot(1) + q_dot(2) + q_dot(3)) + 2*cos(q(1) + q(2))*(q_dot(1) + q_dot(2))))/8 - (m*sin(conj(q(1)) + conj(q(2)))*abs(l)^2*(cos(q(1) + q(2)) + 2*cos(q(1))))/4 + (m*cos(conj(q(1)) + conj(q(2)))*abs(l)^2*(sin(q(1) + q(2)) + 2*sin(q(1))))/4 - (m*abs(l)^2*(cos(conj(q(1)) + conj(q(2)) + conj(q(3))) + 2*cos(conj(q(1)) + conj(q(2))))*(sin(q(1) + q(2) + q(3)) + 2*sin(q(1) + q(2))))/4 + (m*abs(l)^2*(cos(q(1) + q(2) + q(3)) + 2*cos(q(1) + q(2)))*(sin(conj(q(1)) + conj(q(2)) + conj(q(3))) + 2*sin(conj(q(1)) + conj(q(2)))))/4 + (m*cos(conj(q(1)) + conj(q(2)))*sin(q(1) + q(2))*abs(l)^2*(conj(q_dot(1)) + conj(q_dot(2))))/8 - (m*sin(conj(q(1)) + conj(q(2)))*cos(q(1) + q(2))*abs(l)^2*(conj(q_dot(1)) + conj(q_dot(2))))/8 - (m*cos(conj(q(1)) + conj(q(2)))*sin(q(1) + q(2))*abs(l)^2*(q_dot(1) + q_dot(2)))/8 + (m*sin(conj(q(1)) + conj(q(2)))*cos(q(1) + q(2))*abs(l)^2*(q_dot(1) + q_dot(2)))/8,                                                                                                                                                                                                                                                                                                                       (m*abs(l)^2*(2*sin(conj(q(1)) - q(2) - q(3) - q(1) + conj(q(2)))*(q_dot(1) + q_dot(2) + q_dot(3) - conj(q_dot(1)) - conj(q_dot(2))) + sin(conj(q(1)) - q(2) - q(3) - q(1) + conj(q(2)) + conj(q(3)))*(q_dot(1) + q_dot(2) + q_dot(3) - conj(q_dot(1)) - conj(q_dot(2)) - conj(q_dot(3)))))/8 + (m*abs(l)^2*sin(conj(q(1)) - q(2) - q(3) - q(1) + conj(q(2))))/4 + (m*cos(conj(q(1)) + conj(q(2)) + conj(q(3)))*abs(l)^2*(sin(q(1) + q(2) + q(3)) + 2*sin(q(1) + q(2)) + 2*sin(q(1))))/4 - (m*sin(q(1) + q(2) + q(3))*abs(l)^2*(cos(conj(q(1)) + conj(q(2)) + conj(q(3))) + 2*cos(conj(q(1)) + conj(q(2)))))/4 + (m*cos(q(1) + q(2) + q(3))*abs(l)^2*(sin(conj(q(1)) + conj(q(2)) + conj(q(3))) + 2*sin(conj(q(1)) + conj(q(2)))))/4 - (m*sin(conj(q(1)) + conj(q(2)) + conj(q(3)))*abs(l)^2*(cos(q(1) + q(2) + q(3)) + 2*cos(q(1) + q(2)) + 2*cos(q(1))))/4;
                                                                                                                                                                                                                                                                                                                                                                                                                                                                                                                                                                                                                                                                                                                                                                                                      (m*sin(conj(q(1)) - q(2) - q(3) - q(1))*abs(l)^2)/4 + (m*abs(l)^2*(2*sin(conj(q(1)) - q(2) - q(3) - q(1)) + 2*sin(conj(q(1)) - q(2) - q(3) - q(1) + conj(q(2)))))/8 + (m*abs(l)^2*sin(conj(q(1)) - q(2) - q(3) - q(1) + conj(q(2))))/4 - (m*abs(l)^2*sin(conj(q(1)) - q(2) - q(1) + conj(q(2)) + conj(q(3))))/4 + (m*cos(conj(q(1)) + conj(q(2)) + conj(q(3)))*abs(l)^2*(sin(q(1) + q(2) + q(3)) + 2*sin(q(1) + q(2)) + 2*sin(q(1))))/8 - (m*sin(q(1) + q(2) + q(3))*abs(l)^2*(2*cos(conj(q(1))) + cos(conj(q(1)) + conj(q(2)) + conj(q(3))) + 2*cos(conj(q(1)) + conj(q(2)))))/8 + (m*cos(q(1) + q(2) + q(3))*abs(l)^2*(2*sin(conj(q(1))) + sin(conj(q(1)) + conj(q(2)) + conj(q(3))) + 2*sin(conj(q(1)) + conj(q(2)))))/8 + (m*sin(conj(q(1)) + conj(q(2)) + conj(q(3)))*abs(l)^2*(cos(q(1) + q(2) + q(3))*(q_dot(1) + q_dot(2) + q_dot(3)) + 2*cos(q(1) + q(2))*(q_dot(1) + q_dot(2)) + 2*q_dot(1)*cos(q(1))))/8 - (m*cos(conj(q(1)) + conj(q(2)) + conj(q(3)))*abs(l)^2*(sin(q(1) + q(2) + q(3))*(q_dot(1) + q_dot(2) + q_dot(3)) + 2*sin(q(1) + q(2))*(q_dot(1) + q_dot(2)) + 2*q_dot(1)*sin(q(1))))/8 - (m*sin(conj(q(1)) + conj(q(2)) + conj(q(3)))*abs(l)^2*(cos(q(1) + q(2) + q(3)) + 2*cos(q(1) + q(2)) + 2*cos(q(1))))/8 - (m*sin(conj(q(1)) + conj(q(2)) + conj(q(3)))*abs(l)^2*(cos(q(1) + q(2) + q(3)) + 2*cos(q(1) + q(2)) + 2*cos(q(1)))*(conj(q_dot(1)) + conj(q_dot(2)) + conj(q_dot(3))))/8 + (m*cos(conj(q(1)) + conj(q(2)) + conj(q(3)))*abs(l)^2*(sin(q(1) + q(2) + q(3)) + 2*sin(q(1) + q(2)) + 2*sin(q(1)))*(conj(q_dot(1)) + conj(q_dot(2)) + conj(q_dot(3))))/8,                                                                                                                                                                                                                                                                                                                                                                                                                                                                                                                                                                                                                                                                                                                                                                                                            (m*abs(l)^2*sin(conj(q(1)) - q(2) - q(3) - q(1) + conj(q(2))))/4 + (m*cos(conj(q(1)) + conj(q(2)) + conj(q(3)))*abs(l)^2*(sin(q(1) + q(2) + q(3)) + 2*sin(q(1) + q(2)) + 2*sin(q(1))))/4 + (m*sin(conj(q(1)) + conj(q(2)) + conj(q(3)))*abs(l)^2*(cos(q(1) + q(2) + q(3))*(q_dot(1) + q_dot(2) + q_dot(3)) + 2*cos(q(1) + q(2))*(q_dot(1) + q_dot(2))))/8 - (m*cos(conj(q(1)) + conj(q(2)) + conj(q(3)))*abs(l)^2*(sin(q(1) + q(2) + q(3))*(q_dot(1) + q_dot(2) + q_dot(3)) + 2*sin(q(1) + q(2))*(q_dot(1) + q_dot(2))))/8 - (m*sin(q(1) + q(2) + q(3))*abs(l)^2*(cos(conj(q(1)) + conj(q(2)) + conj(q(3))) + 2*cos(conj(q(1)) + conj(q(2)))))/4 + (m*cos(q(1) + q(2) + q(3))*abs(l)^2*(sin(conj(q(1)) + conj(q(2)) + conj(q(3))) + 2*sin(conj(q(1)) + conj(q(2)))))/4 - (m*sin(conj(q(1)) + conj(q(2)) + conj(q(3)))*abs(l)^2*(cos(q(1) + q(2) + q(3)) + 2*cos(q(1) + q(2)) + 2*cos(q(1))))/4 - (m*sin(conj(q(1)) + conj(q(2)) + conj(q(3)))*abs(l)^2*(cos(q(1) + q(2) + q(3)) + 2*cos(q(1) + q(2)))*(conj(q_dot(1)) + conj(q_dot(2)) + conj(q_dot(3))))/8 + (m*cos(conj(q(1)) + conj(q(2)) + conj(q(3)))*abs(l)^2*(sin(q(1) + q(2) + q(3)) + 2*sin(q(1) + q(2)))*(conj(q_dot(1)) + conj(q_dot(2)) + conj(q_dot(3))))/8,                                                                                                                                                                                                                                                                                                                                                            (m*sin(conj(q(1)) - q(2) - q(3) - q(1) + conj(q(2)) + conj(q(3)))*abs(l)^2*(q_dot(1) + q_dot(2) + q_dot(3) - conj(q_dot(1)) - conj(q_dot(2)) - conj(q_dot(3))))/8 + (m*cos(conj(q(1)) + conj(q(2)) + conj(q(3)))*abs(l)^2*(sin(q(1) + q(2) + q(3)) + 2*sin(q(1) + q(2)) + 2*sin(q(1))))/4 + (m*cos(q(1) + q(2) + q(3))*sin(conj(q(1)) + conj(q(2)) + conj(q(3)))*abs(l)^2)/2 - (m*sin(q(1) + q(2) + q(3))*cos(conj(q(1)) + conj(q(2)) + conj(q(3)))*abs(l)^2)/2 - (m*sin(conj(q(1)) + conj(q(2)) + conj(q(3)))*abs(l)^2*(cos(q(1) + q(2) + q(3)) + 2*cos(q(1) + q(2))))/4 + (m*cos(conj(q(1)) + conj(q(2)) + conj(q(3)))*abs(l)^2*(sin(q(1) + q(2) + q(3)) + 2*sin(q(1) + q(2))))/4 - (m*sin(conj(q(1)) + conj(q(2)) + conj(q(3)))*abs(l)^2*(cos(q(1) + q(2) + q(3)) + 2*cos(q(1) + q(2)) + 2*cos(q(1))))/4];

== matlab function Final_Project_v3b/Dynamics Block/G Matrix (set to zero) ==
  data: qqd input; G output; l parameter; m parameter
function G = fcn(qqd,l,m)

q=[qqd(7) qqd(8) qqd(9)];

g=[0 9.81 0]; %gravity acceleration along y


Jp1=[-(l/2)*sin(q(1)) 0 0; (l/2)*cos(q(1)) 0 0; 0 0 0];
Jo1=[0 0 0; 0 0 0; 1 0 0];

Jp2=[-l*sin(q(1))-(l/2)*sin(q(1)+q(2)) -(l/2)*sin(q(1)+q(2)) 0 ;    l*cos(q(1))+(l/2)*cos(q(1)+q(2)) (l/2)*cos(q(1)+q(2)) 0; 0 0 0];
Jo2=[0 0 0; 0 0 0; 1 1 0];

Jp3=[-l*sin(q(1))-l*sin(q(1)+q(2))-(l/2)*sin(q(1)+q(2)+q(3)) -l*sin(q(1)+q(2))-(l/2)*sin(q(1)+q(2)+q(3)) -(l/2)*sin(q(1)+q(2)+q(3)); l*cos(q(1))+(l)*cos(q(1)+q(2))+(l/2)*cos(q(1)+q(2)+q(3)) l*cos(q(1)+q(2))+(l/2)*cos(q(1)+q(2)+q(3)) (l/2)*cos(q(1)+q(2)+q(3)); 0 0 0];
Jo3=[0 0 0; 0 0 0; 1 1 1];

G1=m*(g)*Jp1+m*(g)*Jp2+m*(g)*Jp3;

%G=G1.';

G=[0;0;0];
